simulink model "MPC_Extended_Plant_Simulink"  (R2023b)
settings: Solver=ode4  StartTime=0.0  StopTime=20  FixedStep=1e-3  RelTol=1e-3
values from neighbouring files (symbols this model uses):
  controller_choice = input('Select MPC controller order (1, 2, or 3): ')    [MPC_Extended_Plant.m]    (also in P1.mat = 1; P2.mat = 2; P3.mat = 3)
  init =     [P1.mat]    (also in P2.mat; P3.mat)
  input =     [P1.mat]    (also in P2.mat; P3.mat)
  Np = 40    [MPC_Extended_Plant.m]    (also in P1.mat = 5; P2.mat = 5; P3.mat = 5)
  par =     [P1.mat]    (also in P2.mat; P3.mat)
  Ts = 0.01    [MPC_Extended_Plant.m]    (also in P1.mat; P2.mat; P3.mat)
  V_ref = 16.6666666667    [P1.mat]    (also in P2.mat; P3.mat; veh_parameters.m)
undefined symbols (not defined in the file or in its folder): data
libraries: simulink x12
(part 2 of 2)

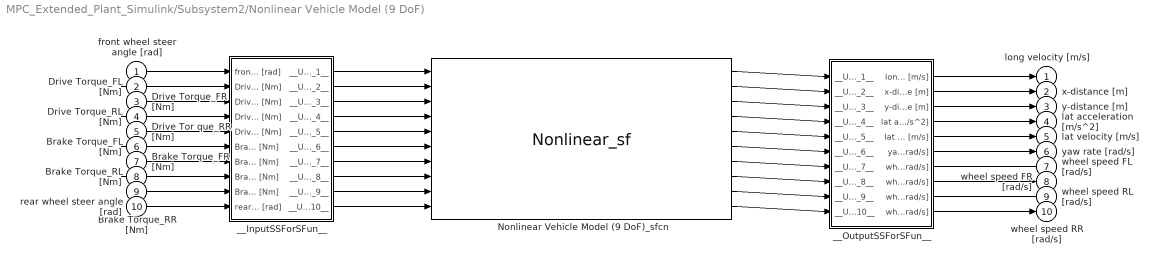
== system MPC_Extended_Plant_Simulink/Subsystem2/Nonlinear Vehicle Model (9 DoF) ==
  front wheel steer angle [rad] : Inport
  Drive Torque_FL [Nm] : Inport  Port=2
  Drive Torque_FR [Nm] : Inport  Port=3
  Drive Torque_RL [Nm] : Inport  Port=4
  Drive Tor	que_RR [Nm] : Inport  Port=5
  Brake Torque_FL [Nm] : Inport  Port=6
  Brake Torque_FR [Nm] : Inport  Port=7
  Brake Torque_RL [Nm] : Inport  Port=8
  Brake Torque_RR [Nm] : Inport  Port=9
  rear wheel steer angle [rad] : Inport  Port=10
  Nonlinear Vehicle Model (9 DoF)_sfcn : S-Function  FunctionName=Nonlinear_sf  SFunctionModules=""  SFunctionDeploymentMode=off  EnableBusSupport=off  mask{rtw_sf_name=Nonlinear_sf, showVar=off}
      mask prompts: rtw_sf_name "Simulink:masks:GenSFuncName_MP"; showVar "Simulink:masks:GenSFuncShowModuleList_MP"
      mask help: Simulink:masks:GenSFuncDesc_MD
      mask init: same as MPC_Extended_Plant_Simulink/Subsystem/Nonlinear Vehicle Model (9 DoF)/Nonlinear Vehicle Model (9 DoF)_sfcn
      settings: CopyFcn=|
      | if ~strcmp(get_param(gcb,'Linkstatus'),'none') && ...
      | ~strcmp(get_param(gcb,'Linkstatus'),'implicit')
      |   set_param(gcb,'LinkStatus','none');
      | end
      mask Help: eval('feval(''rtwprivate'',''rtwhelpview'',''rtw_sfcn_block'')');
      mask Display:
      | port_label('input',1,'front wheel steer angle [rad]');
      | port_label('input',2,'Drive Torque_FL [Nm]');
      | port_label('input',3,'Drive Torque_FR [Nm]');
      | port_label('input',4,'Drive Torque_RL [Nm]');
      | port_label('input',5,'Drive Tor	que_RR [Nm]');
      | port_label('input',6,'Brake Torque_FL [Nm]');
      | port_label('input',7,'Brake Torque_FR [Nm]');
      | port_label('input',8,'Brake Torque_RL [Nm]');
      | port_label('input',9,'Brake Torque_RR [Nm]');
      | port_label('input',10,'rear wheel steer angle [rad]');
      | port_label('output',1,'long velocity [m/s]');
      | port_label('output',2,'x-distance [m]');
      | port_label('output',3,'y-distance [m]');
      | port_label('output',4,'lat acceleration [m/s^2]');
      | port_label('output',5,'lat velocity [m/s]');
      | port_label('output',6,'yaw rate [rad/s]');
      | port_label('output',7,'wheel speed FL [rad/s]');
      | port_label('output',8,'wheel speed FR [rad/s]');
      | port_label('output',9,'wheel speed RL [rad/s]');
      | port_label('output',10,'wheel speed RR [rad/s]');
  __InputSSForSFun__ : Subsystem
  __OutputSSForSFun__ : Subsystem
  long velocity [m/s] : Outport  VectorParamsAs1DForOutWhenUnconnected=off
  x-distance [m] : Outport  Port=2  VectorParamsAs1DForOutWhenUnconnected=off
  y-distance [m] : Outport  Port=3  VectorParamsAs1DForOutWhenUnconnected=off
  lat acceleration [m/s^2] : Outport  Port=4  VectorParamsAs1DForOutWhenUnconnected=off
  lat velocity [m/s] : Outport  Port=5  VectorParamsAs1DForOutWhenUnconnected=off
  yaw rate [rad/s] : Outport  Port=6  VectorParamsAs1DForOutWhenUnconnected=off
  wheel speed FL [rad/s] : Outport  Port=7  VectorParamsAs1DForOutWhenUnconnected=off
  wheel speed FR [rad/s] : Outport  Port=8  VectorParamsAs1DForOutWhenUnconnected=off
  wheel speed RL [rad/s] : Outport  Port=9  VectorParamsAs1DForOutWhenUnconnected=off
  wheel speed RR [rad/s] : Outport  Port=10  VectorParamsAs1DForOutWhenUnconnected=off
  wires:
  front wheel steer angle [rad]/1 -> __InputSSForSFun__/1(front wheel steer angle [rad])
  Drive Torque_FL [Nm]/1 -> __InputSSForSFun__/2(Drive Torque_FL [Nm])
  Drive Torque_FR [Nm]/1 -> __InputSSForSFun__/3(Drive Torque_FR [Nm])
  Drive Torque_RL [Nm]/1 -> __InputSSForSFun__/4(Drive Torque_RL [Nm])
  Drive Tor	que_RR [Nm]/1 -> __InputSSForSFun__/5(Drive Tor	que_RR [Nm])
  Brake Torque_FL [Nm]/1 -> __InputSSForSFun__/6(Brake Torque_FL [Nm])
  Brake Torque_FR [Nm]/1 -> __InputSSForSFun__/7(Brake Torque_FR [Nm])
  Brake Torque_RL [Nm]/1 -> __InputSSForSFun__/8(Brake Torque_RL [Nm])
  Brake Torque_RR [Nm]/1 -> __InputSSForSFun__/9(Brake Torque_RR [Nm])
  rear wheel steer angle [rad]/1 -> __InputSSForSFun__/10(rear wheel steer angle [rad])
  __InputSSForSFun__/1(__UniqueOutportName__1__) -> Nonlinear Vehicle Model (9 DoF)_sfcn/1
  __InputSSForSFun__/2(__UniqueOutportName__2__) -> Nonlinear Vehicle Model (9 DoF)_sfcn/2
  __InputSSForSFun__/3(__UniqueOutportName__3__) -> Nonlinear Vehicle Model (9 DoF)_sfcn/3
  __InputSSForSFun__/4(__UniqueOutportName__4__) -> Nonlinear Vehicle Model (9 DoF)_sfcn/4
  __InputSSForSFun__/5(__UniqueOutportName__5__) -> Nonlinear Vehicle Model (9 DoF)_sfcn/5
  __InputSSForSFun__/6(__UniqueOutportName__6__) -> Nonlinear Vehicle Model (9 DoF)_sfcn/6
  __InputSSForSFun__/7(__UniqueOutportName__7__) -> Nonlinear Vehicle Model (9 DoF)_sfcn/7
  __InputSSForSFun__/8(__UniqueOutportName__8__) -> Nonlinear Vehicle Model (9 DoF)_sfcn/8
  __InputSSForSFun__/9(__UniqueOutportName__9__) -> Nonlinear Vehicle Model (9 DoF)_sfcn/9
  __InputSSForSFun__/10(__UniqueOutportName__10__) -> Nonlinear Vehicle Model (9 DoF)_sfcn/10
  Nonlinear Vehicle Model (9 DoF)_sfcn/1 -> __OutputSSForSFun__/1(__UniqueInportName__1__)
  Nonlinear Vehicle Model (9 DoF)_sfcn/2 -> __OutputSSForSFun__/2(__UniqueInportName__2__)
  Nonlinear Vehicle Model (9 DoF)_sfcn/3 -> __OutputSSForSFun__/3(__UniqueInportName__3__)
  Nonlinear Vehicle Model (9 DoF)_sfcn/4 -> __OutputSSForSFun__/4(__UniqueInportName__4__)
  Nonlinear Vehicle Model (9 DoF)_sfcn/5 -> __OutputSSForSFun__/5(__UniqueInportName__5__)
  Nonlinear Vehicle Model (9 DoF)_sfcn/6 -> __OutputSSForSFun__/6(__UniqueInportName__6__)
  Nonlinear Vehicle Model (9 DoF)_sfcn/7 -> __OutputSSForSFun__/7(__UniqueInportName__7__)
  Nonlinear Vehicle Model (9 DoF)_sfcn/8 -> __OutputSSForSFun__/8(__UniqueInportName__8__)
  Nonlinear Vehicle Model (9 DoF)_sfcn/9 -> __OutputSSForSFun__/9(__UniqueInportName__9__)
  Nonlinear Vehicle Model (9 DoF)_sfcn/10 -> __OutputSSForSFun__/10(__UniqueInportName__10__)
  __OutputSSForSFun__/1(long velocity [m/s]) -> long velocity [m/s]/1
  __OutputSSForSFun__/2(x-distance [m]) -> x-distance [m]/1
  __OutputSSForSFun__/3(y-distance [m]) -> y-distance [m]/1
  __OutputSSForSFun__/4(lat acceleration [m/s^2]) -> lat acceleration [m/s^2]/1
  __OutputSSForSFun__/5(lat velocity [m/s]) -> lat velocity [m/s]/1
  __OutputSSForSFun__/6(yaw rate [rad/s]) -> yaw rate [rad/s]/1
  __OutputSSForSFun__/7(wheel speed FL [rad/s]) -> wheel speed FL [rad/s]/1
  __OutputSSForSFun__/8(wheel speed FR [rad/s]) -> wheel speed FR [rad/s]/1
  __OutputSSForSFun__/9(wheel speed RL [rad/s]) -> wheel speed RL [rad/s]/1
  __OutputSSForSFun__/10(wheel speed RR [rad/s]) -> wheel speed RR [rad/s]/1

== system MPC_Extended_Plant_Simulink/Subsystem2/Regerence Generator ==
  note: yawr_ref
  note: nonlinear response
  note: delta
  note: u
  steering wheel angle [rad] : Inport
  long velocity [m/s] : Inport  Port=2
  MATLAB Function : MATLAB Function  TreatAsAtomicUnit=on
  MATLAB Function1 : MATLAB Function  TreatAsAtomicUnit=on
  Transfer Fcn : TransferFcn  Numerator=[par.wn^2*par.tau par.wn^2]  Denominator=[1 2*par.kseta*par.wn par.wn^2]
  steering ratio : Gain  Gain=1/ par.i_steer
  reference yaw rate [rad/s] : Outport  VectorParamsAs1DForOutWhenUnconnected=off
  wires:
  steering wheel angle [rad]/1 -> steering ratio/1
  steering ratio/1 -> MATLAB Function/1(delta)
  long velocity [m/s]/1 -> MATLAB Function1/2(u), MATLAB Function/2(u)
  MATLAB Function/1(yawr_ss) -> MATLAB Function1/1(yawr_ss)
  MATLAB Function1/1(yawr_sat) -> Transfer Fcn/1
  Transfer Fcn/1 -> reference yaw rate [rad/s]/1

== system MPC_Extended_Plant_Simulink/Subsystem2/Target Speed to Reach ==
  actual speed [m/s] : Inport
  " " : Lookup_n-D  NumberOfTableDimensions=1  BreakpointsForDimension1="[-10  0  10 30]"  IndexSearchMethod=Linear search  Table=[0.1 0.1 1 1]  ExtrapMethod=Clip  RemoveProtectionInput=on  UseLastTableValue=on  RndMeth=Simplest
  Add : Sum  Inputs=+-
  Add1 : Sum
  Gain : Gain  Gain=1000
  Gain1 : Gain  Gain=10
  Ground3 : Ground
  Integrator1 : Integrator  LimitOutput=on  UpperSaturationLimit=0.1  LowerSaturationLimit=-0.1
  Product : Product  RndMeth=Zero
  Product1 : Product  RndMeth=Zero
  Ramp6 : simulink/Sources/Ramp  slope=1  start=0  InitialOutput=0
  Saturation : Saturate  UpperLimit=1  LowerLimit=0
  Switch : Switch  Criteria=u2 > Threshold  Threshold=8  SaturateOnIntegerOverflow=off  InputSameDT=off
  low-pass (1 Hz) : TransferFcn  Denominator=[1/(2*pi) 1]
  "target pre-maneuver speed [m/s] " : Constant  Value=V_ref
  Drive torque [Nm] : Outport
  wires:
  actual speed [m/s]/1 -> low-pass (1 Hz)/1, Add/2
  "target pre-maneuver speed [m/s] "/1 -> Add/1
  Gain1/1 -> Integrator1/1
  Product/1 -> Add1/1
  Add/1 -> Product/1, Product1/1
  Product1/1 -> Gain1/1
  " "/1 -> Product1/2, Product/2
  low-pass (1 Hz)/1 -> " "/1
  Add1/1 -> Saturation/1
  Integrator1/1 -> Add1/2
  Ramp6/1 -> Switch/2
  Switch/1 -> Gain/1
  Ground3/1 -> Switch/1
  Saturation/1 -> Switch/3
  Gain/1 -> Drive torque [Nm]/1

== system MPC_Extended_Plant_Simulink/Subsystem2/steering system ==
  steering wheel angle [rad] : Inport
  Delay : TransportDelay  DelayTime=par.teta_ss
  Steering Dynamics : TransferFcn  Numerator=[par.wn_ss^2]  Denominator=[1 2*par.zeta_ss*par.wn_ss par.wn_ss^2]
  steering ratio : Gain  Gain=1/ par.i_steer
  wheel steer angle [rad] : Outport  VectorParamsAs1DForOutWhenUnconnected=off
  wires:
  steering wheel angle [rad]/1 -> steering ratio/1
  Delay/1 -> Steering Dynamics/1
  steering ratio/1 -> Delay/1
  Steering Dynamics/1 -> wheel steer angle [rad]/1

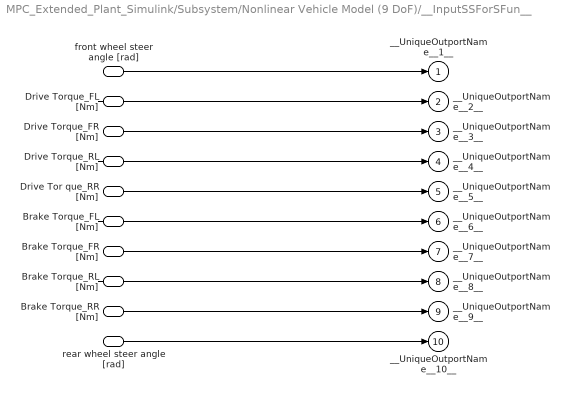
== system MPC_Extended_Plant_Simulink/Subsystem/Nonlinear Vehicle Model (9 DoF)/__InputSSForSFun__ ==
  front wheel steer angle [rad] : Inport
  Drive Torque_FL [Nm] : Inport  Port=2
  Drive Torque_FR [Nm] : Inport  Port=3
  Drive Torque_RL [Nm] : Inport  Port=4
  Drive Tor	que_RR [Nm] : Inport  Port=5
  Brake Torque_FL [Nm] : Inport  Port=6
  Brake Torque_FR [Nm] : Inport  Port=7
  Brake Torque_RL [Nm] : Inport  Port=8
  Brake Torque_RR [Nm] : Inport  Port=9
  rear wheel steer angle [rad] : Inport  Port=10
  __UniqueOutportName__1__ : Outport
  __UniqueOutportName__2__ : Outport  Port=2
  __UniqueOutportName__3__ : Outport  Port=3
  __UniqueOutportName__4__ : Outport  Port=4
  __UniqueOutportName__5__ : Outport  Port=5
  __UniqueOutportName__6__ : Outport  Port=6
  __UniqueOutportName__7__ : Outport  Port=7
  __UniqueOutportName__8__ : Outport  Port=8
  __UniqueOutportName__9__ : Outport  Port=9
  __UniqueOutportName__10__ : Outport  Port=10
  wires:
  front wheel steer angle [rad]/1 -> __UniqueOutportName__1__/1
  Drive Torque_FL [Nm]/1 -> __UniqueOutportName__2__/1
  Drive Torque_FR [Nm]/1 -> __UniqueOutportName__3__/1
  Drive Torque_RL [Nm]/1 -> __UniqueOutportName__4__/1
  Drive Tor	que_RR [Nm]/1 -> __UniqueOutportName__5__/1
  Brake Torque_FL [Nm]/1 -> __UniqueOutportName__6__/1
  Brake Torque_FR [Nm]/1 -> __UniqueOutportName__7__/1
  Brake Torque_RL [Nm]/1 -> __UniqueOutportName__8__/1
  Brake Torque_RR [Nm]/1 -> __UniqueOutportName__9__/1
  rear wheel steer angle [rad]/1 -> __UniqueOutportName__10__/1

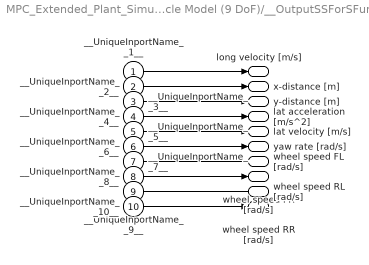
== system MPC_Extended_Plant_Simulink/Subsystem/Nonlinear Vehicle Model (9 DoF)/__OutputSSForSFun__ ==
  __UniqueInportName__1__ : Inport
  __UniqueInportName__2__ : Inport  Port=2
  __UniqueInportName__3__ : Inport  Port=3
  __UniqueInportName__4__ : Inport  Port=4
  __UniqueInportName__5__ : Inport  Port=5
  __UniqueInportName__6__ : Inport  Port=6
  __UniqueInportName__7__ : Inport  Port=7
  __UniqueInportName__8__ : Inport  Port=8
  __UniqueInportName__9__ : Inport  Port=9
  __UniqueInportName__10__ : Inport  Port=10
  long velocity [m/s] : Outport  VectorParamsAs1DForOutWhenUnconnected=off
  x-distance [m] : Outport  Port=2  VectorParamsAs1DForOutWhenUnconnected=off
  y-distance [m] : Outport  Port=3  VectorParamsAs1DForOutWhenUnconnected=off
  lat acceleration [m/s^2] : Outport  Port=4  VectorParamsAs1DForOutWhenUnconnected=off
  lat velocity [m/s] : Outport  Port=5  VectorParamsAs1DForOutWhenUnconnected=off
  yaw rate [rad/s] : Outport  Port=6  VectorParamsAs1DForOutWhenUnconnected=off
  wheel speed FL [rad/s] : Outport  Port=7  VectorParamsAs1DForOutWhenUnconnected=off
  wheel speed FR [rad/s] : Outport  Port=8  VectorParamsAs1DForOutWhenUnconnected=off
  wheel speed RL [rad/s] : Outport  Port=9  VectorParamsAs1DForOutWhenUnconnected=off
  wheel speed RR [rad/s] : Outport  Port=10  VectorParamsAs1DForOutWhenUnconnected=off
  wires:
  __UniqueInportName__1__/1 -> long velocity [m/s]/1
  __UniqueInportName__2__/1 -> x-distance [m]/1
  __UniqueInportName__3__/1 -> y-distance [m]/1
  __UniqueInportName__4__/1 -> lat acceleration [m/s^2]/1
  __UniqueInportName__5__/1 -> lat velocity [m/s]/1
  __UniqueInportName__6__/1 -> yaw rate [rad/s]/1
  __UniqueInportName__7__/1 -> wheel speed FL [rad/s]/1
  __UniqueInportName__8__/1 -> wheel speed FR [rad/s]/1
  __UniqueInportName__9__/1 -> wheel speed RL [rad/s]/1
  __UniqueInportName__10__/1 -> wheel speed RR [rad/s]/1

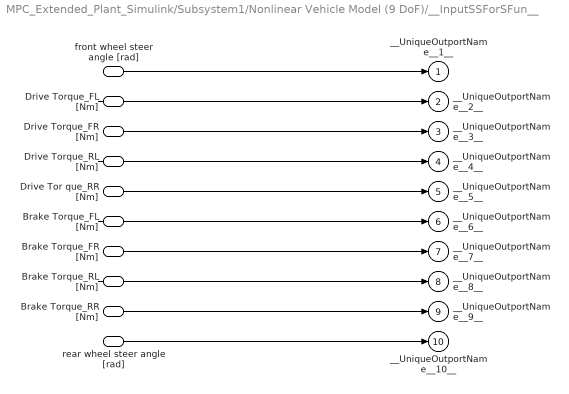
== system MPC_Extended_Plant_Simulink/Subsystem1/Nonlinear Vehicle Model (9 DoF)/__InputSSForSFun__ ==
  front wheel steer angle [rad] : Inport
  Drive Torque_FL [Nm] : Inport  Port=2
  Drive Torque_FR [Nm] : Inport  Port=3
  Drive Torque_RL [Nm] : Inport  Port=4
  Drive Tor	que_RR [Nm] : Inport  Port=5
  Brake Torque_FL [Nm] : Inport  Port=6
  Brake Torque_FR [Nm] : Inport  Port=7
  Brake Torque_RL [Nm] : Inport  Port=8
  Brake Torque_RR [Nm] : Inport  Port=9
  rear wheel steer angle [rad] : Inport  Port=10
  __UniqueOutportName__1__ : Outport
  __UniqueOutportName__2__ : Outport  Port=2
  __UniqueOutportName__3__ : Outport  Port=3
  __UniqueOutportName__4__ : Outport  Port=4
  __UniqueOutportName__5__ : Outport  Port=5
  __UniqueOutportName__6__ : Outport  Port=6
  __UniqueOutportName__7__ : Outport  Port=7
  __UniqueOutportName__8__ : Outport  Port=8
  __UniqueOutportName__9__ : Outport  Port=9
  __UniqueOutportName__10__ : Outport  Port=10
  wires:
  front wheel steer angle [rad]/1 -> __UniqueOutportName__1__/1
  Drive Torque_FL [Nm]/1 -> __UniqueOutportName__2__/1
  Drive Torque_FR [Nm]/1 -> __UniqueOutportName__3__/1
  Drive Torque_RL [Nm]/1 -> __UniqueOutportName__4__/1
  Drive Tor	que_RR [Nm]/1 -> __UniqueOutportName__5__/1
  Brake Torque_FL [Nm]/1 -> __UniqueOutportName__6__/1
  Brake Torque_FR [Nm]/1 -> __UniqueOutportName__7__/1
  Brake Torque_RL [Nm]/1 -> __UniqueOutportName__8__/1
  Brake Torque_RR [Nm]/1 -> __UniqueOutportName__9__/1
  rear wheel steer angle [rad]/1 -> __UniqueOutportName__10__/1

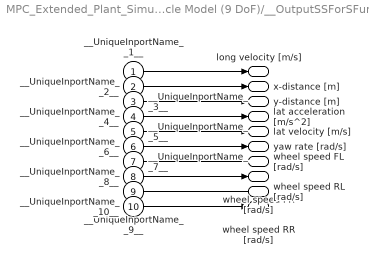
== system MPC_Extended_Plant_Simulink/Subsystem1/Nonlinear Vehicle Model (9 DoF)/__OutputSSForSFun__ ==
  __UniqueInportName__1__ : Inport
  __UniqueInportName__2__ : Inport  Port=2
  __UniqueInportName__3__ : Inport  Port=3
  __UniqueInportName__4__ : Inport  Port=4
  __UniqueInportName__5__ : Inport  Port=5
  __UniqueInportName__6__ : Inport  Port=6
  __UniqueInportName__7__ : Inport  Port=7
  __UniqueInportName__8__ : Inport  Port=8
  __UniqueInportName__9__ : Inport  Port=9
  __UniqueInportName__10__ : Inport  Port=10
  long velocity [m/s] : Outport  VectorParamsAs1DForOutWhenUnconnected=off
  x-distance [m] : Outport  Port=2  VectorParamsAs1DForOutWhenUnconnected=off
  y-distance [m] : Outport  Port=3  VectorParamsAs1DForOutWhenUnconnected=off
  lat acceleration [m/s^2] : Outport  Port=4  VectorParamsAs1DForOutWhenUnconnected=off
  lat velocity [m/s] : Outport  Port=5  VectorParamsAs1DForOutWhenUnconnected=off
  yaw rate [rad/s] : Outport  Port=6  VectorParamsAs1DForOutWhenUnconnected=off
  wheel speed FL [rad/s] : Outport  Port=7  VectorParamsAs1DForOutWhenUnconnected=off
  wheel speed FR [rad/s] : Outport  Port=8  VectorParamsAs1DForOutWhenUnconnected=off
  wheel speed RL [rad/s] : Outport  Port=9  VectorParamsAs1DForOutWhenUnconnected=off
  wheel speed RR [rad/s] : Outport  Port=10  VectorParamsAs1DForOutWhenUnconnected=off
  wires:
  __UniqueInportName__1__/1 -> long velocity [m/s]/1
  __UniqueInportName__2__/1 -> x-distance [m]/1
  __UniqueInportName__3__/1 -> y-distance [m]/1
  __UniqueInportName__4__/1 -> lat acceleration [m/s^2]/1
  __UniqueInportName__5__/1 -> lat velocity [m/s]/1
  __UniqueInportName__6__/1 -> yaw rate [rad/s]/1
  __UniqueInportName__7__/1 -> wheel speed FL [rad/s]/1
  __UniqueInportName__8__/1 -> wheel speed FR [rad/s]/1
  __UniqueInportName__9__/1 -> wheel speed RL [rad/s]/1
  __UniqueInportName__10__/1 -> wheel speed RR [rad/s]/1

== system MPC_Extended_Plant_Simulink/Subsystem2/Nonlinear Vehicle Model (9 DoF)/__InputSSForSFun__ ==
  front wheel steer angle [rad] : Inport
  Drive Torque_FL [Nm] : Inport  Port=2
  Drive Torque_FR [Nm] : Inport  Port=3
  Drive Torque_RL [Nm] : Inport  Port=4
  Drive Tor	que_RR [Nm] : Inport  Port=5
  Brake Torque_FL [Nm] : Inport  Port=6
  Brake Torque_FR [Nm] : Inport  Port=7
  Brake Torque_RL [Nm] : Inport  Port=8
  Brake Torque_RR [Nm] : Inport  Port=9
  rear wheel steer angle [rad] : Inport  Port=10
  __UniqueOutportName__1__ : Outport
  __UniqueOutportName__2__ : Outport  Port=2
  __UniqueOutportName__3__ : Outport  Port=3
  __UniqueOutportName__4__ : Outport  Port=4
  __UniqueOutportName__5__ : Outport  Port=5
  __UniqueOutportName__6__ : Outport  Port=6
  __UniqueOutportName__7__ : Outport  Port=7
  __UniqueOutportName__8__ : Outport  Port=8
  __UniqueOutportName__9__ : Outport  Port=9
  __UniqueOutportName__10__ : Outport  Port=10
  wires:
  front wheel steer angle [rad]/1 -> __UniqueOutportName__1__/1
  Drive Torque_FL [Nm]/1 -> __UniqueOutportName__2__/1
  Drive Torque_FR [Nm]/1 -> __UniqueOutportName__3__/1
  Drive Torque_RL [Nm]/1 -> __UniqueOutportName__4__/1
  Drive Tor	que_RR [Nm]/1 -> __UniqueOutportName__5__/1
  Brake Torque_FL [Nm]/1 -> __UniqueOutportName__6__/1
  Brake Torque_FR [Nm]/1 -> __UniqueOutportName__7__/1
  Brake Torque_RL [Nm]/1 -> __UniqueOutportName__8__/1
  Brake Torque_RR [Nm]/1 -> __UniqueOutportName__9__/1
  rear wheel steer angle [rad]/1 -> __UniqueOutportName__10__/1

== system MPC_Extended_Plant_Simulink/Subsystem2/Nonlinear Vehicle Model (9 DoF)/__OutputSSForSFun__ ==
  __UniqueInportName__1__ : Inport
  __UniqueInportName__2__ : Inport  Port=2
  __UniqueInportName__3__ : Inport  Port=3
  __UniqueInportName__4__ : Inport  Port=4
  __UniqueInportName__5__ : Inport  Port=5
  __UniqueInportName__6__ : Inport  Port=6
  __UniqueInportName__7__ : Inport  Port=7
  __UniqueInportName__8__ : Inport  Port=8
  __UniqueInportName__9__ : Inport  Port=9
  __UniqueInportName__10__ : Inport  Port=10
  long velocity [m/s] : Outport  VectorParamsAs1DForOutWhenUnconnected=off
  x-distance [m] : Outport  Port=2  VectorParamsAs1DForOutWhenUnconnected=off
  y-distance [m] : Outport  Port=3  VectorParamsAs1DForOutWhenUnconnected=off
  lat acceleration [m/s^2] : Outport  Port=4  VectorParamsAs1DForOutWhenUnconnected=off
  lat velocity [m/s] : Outport  Port=5  VectorParamsAs1DForOutWhenUnconnected=off
  yaw rate [rad/s] : Outport  Port=6  VectorParamsAs1DForOutWhenUnconnected=off
  wheel speed FL [rad/s] : Outport  Port=7  VectorParamsAs1DForOutWhenUnconnected=off
  wheel speed FR [rad/s] : Outport  Port=8  VectorParamsAs1DForOutWhenUnconnected=off
  wheel speed RL [rad/s] : Outport  Port=9  VectorParamsAs1DForOutWhenUnconnected=off
  wheel speed RR [rad/s] : Outport  Port=10  VectorParamsAs1DForOutWhenUnconnected=off
  wires:
  __UniqueInportName__1__/1 -> long velocity [m/s]/1
  __UniqueInportName__2__/1 -> x-distance [m]/1
  __UniqueInportName__3__/1 -> y-distance [m]/1
  __UniqueInportName__4__/1 -> lat acceleration [m/s^2]/1
  __UniqueInportName__5__/1 -> lat velocity [m/s]/1
  __UniqueInportName__6__/1 -> yaw rate [rad/s]/1
  __UniqueInportName__7__/1 -> wheel speed FL [rad/s]/1
  __UniqueInportName__8__/1 -> wheel speed FR [rad/s]/1
  __UniqueInportName__9__/1 -> wheel speed RL [rad/s]/1
  __UniqueInportName__10__/1 -> wheel speed RR [rad/s]/1

== matlab function MPC_Extended_Plant_Simulink/Subsystem1/Regerence Generator/MATLAB Function1 ==
  data: yawr_ss input; u input; yawr_sat output; par parameter
function yawr_sat = boundary_conditions(yawr_ss,u,par)
g = par.g;
mu = par.mu;

yawr_max = 0.85*mu*g/u;

if abs(yawr_ss) > abs(yawr_max)
    yawr_sat = sign(yawr_ss)*yawr_max;
else
    yawr_sat = yawr_ss;
end

== matlab function MPC_Extended_Plant_Simulink/Subsystem2/Regerence Generator/MATLAB Function ==
  data: delta input; u input; yawr_ss output; par parameter
function yawr_ss = bicycle_model(delta,u,par)
%Parameters
L = par.L;
g = par.g;
m = par.mass;
K = par.Kus;

%Yaw rate response
yawr_ss = u*delta/(L+K*u^2/g);

== matlab function MPC_Extended_Plant_Simulink/Subsystem/MPC Controller (automatically updated after new code generation)/Shift reference ==
  data: y output; yN input; Np parameter
function y = shift_reference(yN,Np)

y=repmat([yN;0;0;0;0],Np,1)';

end

== matlab function MPC_Extended_Plant_Simulink/Subsystem2/MPC Controller (automatically updated after new code generation)/Shift reference ==
  data: y output; yN input; Np parameter
function y = shift_reference(yN,Np)

y=repmat([yN;0;0;0;0],Np,1)';

end

== matlab function MPC_Extended_Plant_Simulink/Subsystem/MPC Controller (automatically updated after new code generation)/Shift reference1 ==
  data: y output; yN input; Np parameter
function y = shift_reference(yN,Np)

y=repmat(yN,Np+1,1)';

end

== matlab function MPC_Extended_Plant_Simulink/Subsystem2/MPC Controller (automatically updated after new code generation)/Shift reference2 ==
  data: y output; yN input; Np parameter
function y = shift_reference(yN,Np)

y=repmat(yN,Np+1,1)';

end

== matlab function MPC_Extended_Plant_Simulink/Subsystem/Regerence Generator/MATLAB Function ==
  data: delta input; u input; yawr_ss output; par parameter
function yawr_ss = bicycle_model(delta,u,par)
%Parameters
L = par.L;
g = par.g;
m = par.mass;
K = par.Kus;

%Yaw rate response
yawr_ss = u*delta/(L+K*u^2/g);

== matlab function MPC_Extended_Plant_Simulink/Subsystem/Regerence Generator/MATLAB Function1 ==
  data: yawr_ss input; u input; yawr_sat output; par parameter
function yawr_sat = boundary_conditions(yawr_ss,u,par)
g = par.g;
mu = par.mu;

yawr_max = 0.85*mu*g/u;

if abs(yawr_ss) > abs(yawr_max)
    yawr_sat = sign(yawr_ss)*yawr_max;
else
    yawr_sat = yawr_ss;
end

== matlab function MPC_Extended_Plant_Simulink/Subsystem1/MPC Controller (automatically updated after new code generation)/Shift reference ==
  data: y output; yN input; Np parameter
function y = shift_reference(yN,Np)

y=repmat([yN;0;0;0;0],Np,1)';

end

== matlab function MPC_Extended_Plant_Simulink/Subsystem1/MPC Controller (automatically updated after new code generation)/Shift reference2 ==
  data: y output; yN input; Np parameter
function y = shift_reference(yN,Np)

y=repmat(yN,Np+1,1)';

end

== matlab function MPC_Extended_Plant_Simulink/Subsystem2/Regerence Generator/MATLAB Function1 ==
  data: yawr_ss input; u input; yawr_sat output; par parameter
function yawr_sat = boundary_conditions(yawr_ss,u,par)
g = par.g;
mu = par.mu;

yawr_max = 0.85*mu*g/u;

if abs(yawr_ss) > abs(yawr_max)
    yawr_sat = sign(yawr_ss)*yawr_max;
else
    yawr_sat = yawr_ss;
end

== matlab function MPC_Extended_Plant_Simulink/Subsystem1/Regerence Generator/MATLAB Function ==
  data: delta input; u input; yawr_ss output; par parameter
function yawr_ss = bicycle_model(delta,u,par)
%Parameters
L = par.L;
g = par.g;
m = par.mass;
K = par.Kus;

%Yaw rate response
yawr_ss = u*delta/(L+K*u^2/g);
